simulink model "Q1"  (R2018b)
settings: Solver=VariableStepAuto  StartTime=0.0  StopTime=40  RelTol=1e-3
values from neighbouring files (symbols this model uses):
  k = kt(1:length(sys.A))    [questao1.m]    (also in questao3.m = kt(1:length(A)))
  ka = -kt(end)    [questao1.m]    (also in questao3.m)
  sys = ss(G)    [questao1.m]
  x0 = [0 ... (first row only)    [questao1.m]    (also in questao3.m = [v_h1, v_h2])
libraries: simulink x1
settings Model: Creator=bernardo  LastModifiedBy=bernardo

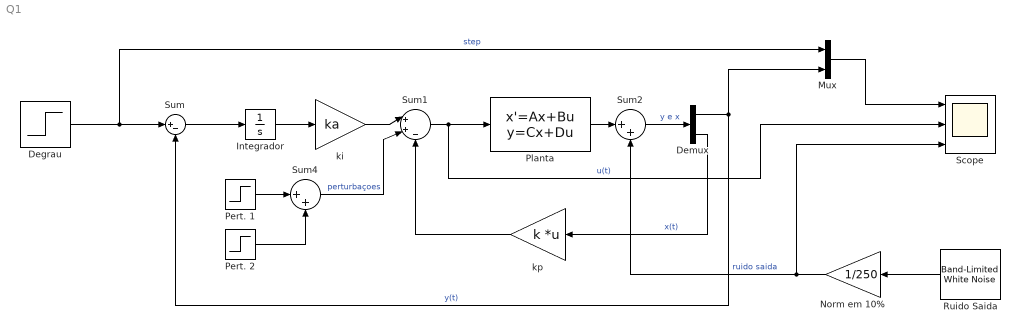
== system Q1 ==
  Degrau : Step  Time=10  SampleTime=0.001
  Demux : Demux  Outputs=[1, length(sys.A)]
  Integrador : Integrator
  Mux : Mux  Inputs=2
  Norm em 10% : Gain  Gain=1/250
  Pert. 1 : Step  Time=20  After=-1/10  SampleTime=0.001
  Pert. 2 : Step  Time=30  After=1/10  SampleTime=0.001
  Planta : StateSpace  A=sys.A  B=sys.B  C=[sys.C; eye( length(sys.A) ) ]  D=[sys.D; zeros( length(sys.A), 1 ) ]  InitialCondition=x0
  Ruido Saida : simulink/Sources/Band-Limited White Noise  Cov=[0.1]  Ts=0.01  seed=[23341]
  Scope : Scope  NumInputPorts=3
  Sum : Sum  Inputs=|+-
  Sum1 : Sum  Inputs=|++-
  Sum2 : Sum  Inputs=|++
  Sum4 : Sum  Inputs=|++
  ki : Gain  Gain=ka
  kp : Gain  Gain=k  Multiplication=Matrix(K*u)
  wires:
  Sum1/1 -> Scope/2, Planta/1  "u(t)"
  kp/1 -> Sum1/3
  Integrador/1 -> ki/1
  ki/1 -> Sum1/1
  Sum/1 -> Integrador/1
  Degrau/1 -> Mux/1, Sum/1  "step"
  Ruido Saida/1 -> Norm em 10%/1
  Norm em 10%/1 -> Scope/3, Sum2/2  "ruido saida"
  Planta/1 -> Sum2/1
  Mux/1 -> Scope/1
  Demux/2 -> kp/1  "x(t)"
  Pert. 1/1 -> Sum4/1
  Pert. 2/1 -> Sum4/2
  Sum4/1 -> Sum1/2  "perturbaçoes"
  Sum2/1 -> Demux/1  "y e x"
  Demux/1 -> Mux/2, Sum/2  "y(t)"
